simulink library "MFBD_lib"  (R2013a)
settings: Solver=ode45  StartTime=0.0  StopTime=10.0  RelTol=1e-3
values from neighbouring files (symbols this model uses):
  DPa0 = 'NA'    [getDataFromNASTRAN.m]
  EV_C = 0    [getDataFromNASTRAN.m]
  LS = 0    [getDataFromNASTRAN.m]
  omega = 0    [getDataFromNASTRAN.m]
  zeta = 'Inf'    [getDataFromNASTRAN.m]
undefined symbols (not defined in the file or in its folder): uev, uls, uw
undefined symbols (not defined in the file): ureal
libraries: RCTblocks x11, cstblocks x2
settings Model: Creator=d.alazard  LastModifiedBy=d.alazard

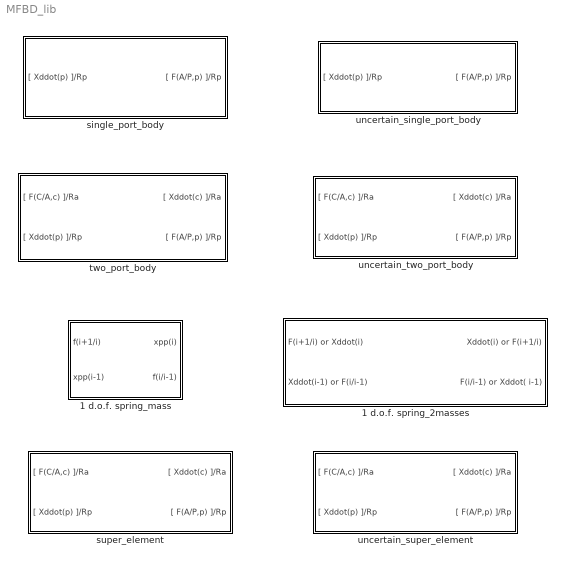
== system MFBD_lib ==
  1 d.o.f. spring_2masses : Subsystem  AncestorBlock=MFBD_lib/super_element  mask{m1=1, m2=1, k=1, c=Direct}
      mask prompts: m1 "Upstream mass: m1 (Kg)"; m2 "Downstream mass: m2 (Kg)"; k "Stiffness: k (N/m)"; c "Direct or Inverse"
      mask init:
      | path(path,'..')
      | if c==1,
      |     MKmodel=Z_elem(m1,k,m2,'d');
      | elseif c==2,
      |     MKmodel=Z_elem(m1,k,m2,'i');
      | elseif c==3,
      |     MKmodel=Z_elem(m1,k,m2,'iu');
      | elseif c==4,
      |     MKmodel=Z_elem(m1,k,m2,'il');
      | end
      mask TypeOptions c: Direct | Inverse | Upper inverse | Lower Inverse
  1 d.o.f. spring_mass : Subsystem  mask{m=0.1, k=2}
      mask prompts: m "Mass"; k "Stiffness"
  "single_port_body " : Subsystem  mask{R_angval=[0 0 0], R_sequence=ZYX, Xi=0, p_gp=1, nf=2, fbdf=file_name, ff06=file_name}
      mask prompts: R_angval "Rotation angles for appendage reference frame at P with respect to parent reference frame"; R_sequence "Rotation sequence for appendage reference frame at P"; Xi "Damping ratio for appendage"; p_gp "Grid point index corresponding to point P of appendage"; nf "No. of modes to be considered"; fbdf "Name of the .bdf file (without extension)"; ff06 "Name of the .f06 file (without extension)"
      mask init:
      | maskStr = get_param(gcb,'MaskValues');
      | R_angrad = R_angval*pi/180;
      | R_seqstr = maskStr{2};
      | dcm_au = angle2dcm(R_angrad(1),R_angrad(2),R_angrad(3),R_seqstr);
      | path(path,'..')
      | a=char(strcat(maskStr{7},'.f06'));
      | b=char(strcat(maskStr{6},'.bdf'));
      | [M, J, xcg, LS, omega, EV_C, zeta, DPa0, cdP, cdC, flagFatal] = ... 
      |     getDataFromNASTRAN(a,b,'f',Xi,p_gp,p_gp,nf);
      mask TypeOptions R_sequence: ZYX | ZYZ | ZXY | ZXZ | YXZ | YXY | YZX | YZY | XYZ | XYX | XZY | XZX
  super_element : Subsystem  AncestorBlock=MFBD_lib/super_element  mask{rho=1, s=1, l1=1, e=1, nu=1, iz=1, iy=1, ipx=1, xi=1, R_angval=[0 0 0], R_sequence=ZYX}
      mask prompts: rho "Material density, rho (kg/m^3)"; s "Beam section area, S (m^2)"; l1 "Length of the beam, L (m)"; e "Modulus of elasticity, E (Pa or N/m^2)"; nu "Poisson's ratio (Range: 0 to 0.5)"; iz "Area moment of inertia along z axis, Izz (m^4)"; iy "Area moment of inertia along y axis, Iyy (m^4)"; ipx "Polar second moment of inertia, Ipx (m^4)"; xi "Damping ratio, xi"; R_angval "Rotation angles for element reference frame at P with respect to parent reference frame"; R_sequence "Rotation sequence for element reference frame at P"
      mask init:
      | maskStr = get_param(gcb,'MaskValues');
      | R_angrad = R_angval*pi/180;
      | R_seqstr = maskStr{11};
      | dcm_eu = angle2dcm(R_angrad(1),R_angrad(2),R_angrad(3),R_seqstr);
      | g=e/(2*(1+nu));
      | path(path,'..')
      | Mm1M=TwoPortBeam(rho,s,l1,e,g,iz,iy,ipx,xi);
      mask TypeOptions R_sequence: ZYX | ZYZ | ZXY | ZXZ | YXZ | YXY | YZX | YZY | XYZ | XYX | XZY | XZX
  two_port_body : Subsystem  mask{R_angval=[0 0 0], R_sequence=ZYX, Xi=0, p_gp=1, C_gp=1, nf=2, fbdf=file_name, ff06=file_name}
      mask prompts: R_angval "Rotation angles for appendage reference frame at P with respect to parent reference frame"; R_sequence "Rotation sequence for appendage reference frame at P"; Xi "Damping ratio for appendage"; p_gp "Grid point index corresponding to point P of appendage"; C_gp "Grid point index corresponding to point C of appendage"; nf "No of modes"; fbdf "Name of the .bdf file (without extension)"; ff06 "Name of the .f06 file (without extension)"
      mask init:
      | maskStr = get_param(gcb,'MaskValues');
      | R_angrad = R_angval*pi/180;
      | R_seqstr = maskStr{2};
      | dcm_au = angle2dcm(R_angrad(1),R_angrad(2),R_angrad(3),R_seqstr);
      | path(path,'..')
      | a=char(strcat(maskStr{8},'.f06'));
      | b=char(strcat(maskStr{7},'.bdf'));
      | [M, J, xcg, LS, omega, EV_C, zeta, DPa0, cdP, cdC, flagFatal] = ... 
      |     getDataFromNASTRAN(a,b,'f',Xi,p_gp,C_gp,nf);
      | 
      | CPvec=cdP-cdC;
      | tauCP=[eye(3) [0 -CPvec(3) CPvec(2);
      |                CPvec(3) 0 -CPvec(1);
      |               -CPvec(2) CPvec(1) 0];
      |               zeros(3) eye(3)];
      mask TypeOptions R_sequence: ZYX | ZYZ | ZXY | ZXZ | YXZ | YXY | YZX | YZY | XYZ | XYX | XZY | XZX
  uncertain_single_port_body : Subsystem  mask{R_angval=[0 0 0], R_sequence=ZYX, Xi=0, p_gp=1, uw_var=0, uls_var=0, nf=2, fbdf=file_name, ff06=file_name}
      mask prompts: R_angval "Rotation angles for appendage reference frame at P with respect to parent reference frame"; R_sequence "Rotation sequence for appendage reference frame at P"; Xi "Damping ratio for appendage"; p_gp "Grid point index corresponding to point P of appendage"; uw_var "Percentage of uncertainity for natural frequencies"; uls_var "Percentage of uncertainity for modal participation factors"; nf "Number of modes"; fbdf "Name of the .bdf file (without extension)"; ff06 "Name of the .f06 file (without extension)"
      mask init:
      | maskStr = get_param(gcb,'MaskValues');
      | R_angrad = R_angval*pi/180;
      | R_seqstr = maskStr{2};
      | dcm_au = angle2dcm(R_angrad(1),R_angrad(2),R_angrad(3),R_seqstr);
      | path(path,'..')
      | a=char(strcat(maskStr{9},'.f06'));
      | b=char(strcat(maskStr{8},'.bdf'));
      | [M, J, xcg, LS, omega, EV_C, zeta, DPa0, cdP, cdC, flagFatal] = ... 
      |     getDataFromNASTRAN(a,b,'f',Xi,p_gp,p_gp,nf);
      | for i=1:size(omega)
      |     uw(i)=eval(['ureal(''uwa' num2str(i) ''',' num2str(omega(i)) ... 
      |         ',''Percentage'',' num2str(uw_var) ')' ]);
      | end
      | 
      | sLS=size(LS);
      | 
      | for i=1:sLS(1)
      |     for j=1:sLS(2)
      |         if(LS(i,j)==0)
      |             uls(i,j)=0;
      |         else
      |         uls(i,j)=eval(['ureal(''ulsa' num2str(i) num2str(j) ''',' num2str(LS(i,j)) ... 
      |         ',''Percentage'',' num2str(uls_var) ')' ]);
      |         end
      |     end
      | end
      mask TypeOptions R_sequence: ZYX | ZYZ | ZXY | ZXZ | YXZ | YXY | YZX | YZY | XYZ | XYX | XZY | XZX
  uncertain_super_element : Subsystem  AncestorBlock=MFBD_lib/super_element  mask{rho=ureal('rho',1,'Percentage',1), s=ureal('S',1,'Percentage',1), l1=ureal('L',1,'Percentage',1), e=ureal('E',1,'Percentage',1), nu=ureal('nu',0.3,'Percentage',1), iz=ureal('Izz',1,'Percentage',1), iy=ureal('Iyy',1,'Percentage',1), ipx=ureal('Ipx',1,'Percentage',1), xi=ureal('xi',1,'Percentage',1), R_angval=[0 0 0], R_sequence=ZYX}
      mask prompts: rho "Material density, rho (kg/m^3)"; s "Beam section area, S (m^2)"; l1 "Length of the beam, L (m)"; e "Modulus of elasticity, E (Pa or N/m^2)"; nu "Poisson's ratio (Range: 0 to 0.5)"; iz "Area moment of inertia along z axis, Izz (m^4)"; iy "Area moment of inertia along y axis, Iyy (m^4)"; ipx "Polar second moment of inertia, Ipx (m^4)"; xi "Damping ratio, xi"; R_angval "Rotation angles for element reference frame at P with respect to parent reference frame"; R_sequence "Rotation sequence for element reference frame at P"
      mask init:
      | maskStr = get_param(gcb,'MaskValues');
      | R_angrad = R_angval*pi/180;
      | R_seqstr = maskStr{11};
      | dcm_eu = angle2dcm(R_angrad(1),R_angrad(2),R_angrad(3),R_seqstr);
      | path(path,'..')
      | g=e/(2*(1+nu));
      | Mm1M=TwoPortBeam(rho,s,l1,e,g,iz,iy,ipx,xi);
      mask TypeOptions R_sequence: ZYX | ZYZ | ZXY | ZXZ | YXZ | YXY | YZX | YZY | XYZ | XYX | XZY | XZX
  uncertain_two_port_body : Subsystem  mask{R_angval=[0 0 0], R_sequence=ZYX, Xi=0, p_gp=1, C_gp=1, uw_var=0, uev_var=0, uls_var=0, nf=2, fbdf=file_name, ff06=file_name}
      mask prompts: R_angval "Rotation angles for appendage reference frame at P with respect to parent reference frame"; R_sequence "Rotation sequence for appendage reference frame at P"; Xi "Damping ratio for appendage"; p_gp "Grid point index corresponding to point P of appendage"; C_gp "Grid point index corresponding to point C of appendage"; uw_var "Percentage of uncertainity for natural frequencies"; uev_var "Percentage of uncertainity for Eigen vectors"; uls_var "Percentage of uncertainity for modal participation factors"; nf "No. of modes"; fbdf "Name of the .bdf file (without extension)"; ff06 "Name of the .f06 file (without extension)"
      mask init:
      | maskStr = get_param(gcb,'MaskValues');
      | R_angrad = R_angval*pi/180;
      | R_seqstr = maskStr{2};
      | dcm_au = angle2dcm(R_angrad(1),R_angrad(2),R_angrad(3),R_seqstr);
      | path(path,'..')
      | a=char(strcat(maskStr{11},'.f06'));
      | b=char(strcat(maskStr{10},'.bdf'));
      | [M, J, xcg, LS, omega, EV_C, zeta, DPa0, cdP, cdC, flagFatal] = ... 
      |     getDataFromNASTRAN(a,b,'f',Xi,p_gp,C_gp,nf);
      | 
      | CPvec=cdP-cdC;
      | tauCP=[eye(3) [0 -CPvec(3) CPvec(2);
      |                CPvec(3) 0 -CPvec(1);
      |               -CPvec(2) CPvec(1) 0];
      |               zeros(3) eye(3)];
      | 
      | for i=1:size(omega)
      |     uw(i)=eval(['ureal(''uwa' num2str(i) ''',' num2str(omega(i)) ... 
      |         ',''Percentage'',' num2str(uw_var) ')' ]);
      | end
      | 
      | sLS=size(LS);
      | sEV=size(EV_C);
      | 
      | for i=1:sLS(1)
      |     for j=1:sLS(2)
      |         if(LS(i,j)==0)
      |             uls(i,j)=0;
      |         else
      |         uls(i,j)=eval(['ureal(''ulsa' num2str(i) num2str(j) ''',' num2str(LS(i,j)) ... 
      |         ',''Percentage'',' num2str(uls_var) ')' ]);
      |         end
      |     end
      | end
      | 
      | for i=1:sEV(1)
      |     for j=1:sEV(2)
      |         if(EV_C(i,j)==0)
      |             uev(i,j)=0;
      |         else
      |         uev(i,j)=eval(['ureal(''ueva' num2str(i) num2str(j) ''',' num2str(EV_C(i,j)) ... 
      |         ',''Percentage'',' num2str(uev_var) ')' ]);
      |         end
      |     end
      | end
      mask TypeOptions R_sequence: ZYX | ZYZ | ZXY | ZXZ | YXZ | YXY | YZX | YZY | XYZ | XYX | XZY | XZX

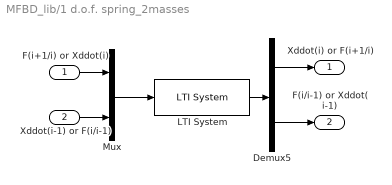
== system MFBD_lib/1 d.o.f. spring_2masses ==
  F(i+1/i) or Xddot(i) : Inport
  Xddot(i-1) or F(i/i-1) : Inport  Port=2
  Demux5 : Demux  Outputs=2
  LTI System : cstblocks/LTI System  sys=MKmodel  IC=[]
  Mux : Mux  Inputs=2
  Xddot(i) or F(i+1/i) : Outport
  F(i/i-1) or Xddot( i-1) : Outport  Port=2
  wires:
  Mux/1 -> LTI System/1
  LTI System/1 -> Demux5/1
  F(i+1/i) or Xddot(i)/1 -> Mux/1
  Xddot(i-1) or F(i/i-1)/1 -> Mux/2
  Demux5/1 -> Xddot(i) or F(i+1/i)/1
  Demux5/2 -> F(i/i-1) or Xddot( i-1)/1

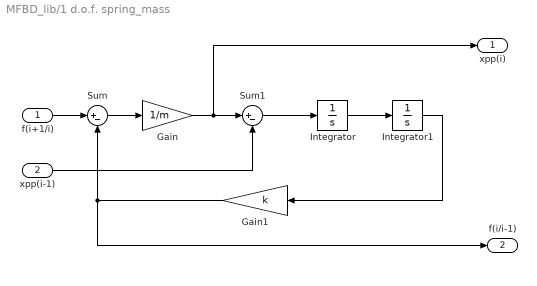
== system MFBD_lib/1 d.o.f. spring_mass ==
  f(i+1/i) : Inport
  xpp(i-1) : Inport  Port=2
  Gain : Gain  Gain=1/m
  Gain1 : Gain  Gain=k
  Integrator : Integrator
  Integrator1 : Integrator
  Sum : Sum  Inputs=|+-
  Sum1 : Sum  Inputs=|+-
  xpp(i) : Outport
  f(i/i-1) : Outport  Port=2
  wires:
  xpp(i-1)/1 -> Sum1/2
  f(i+1/i)/1 -> Sum/1
  Integrator1/1 -> Gain1/1
  Sum1/1 -> Integrator/1
  Integrator/1 -> Integrator1/1
  Sum/1 -> Gain/1
  Gain/1 -> xpp(i)/1, Sum1/1
  Gain1/1 -> f(i/i-1)/1, Sum/2

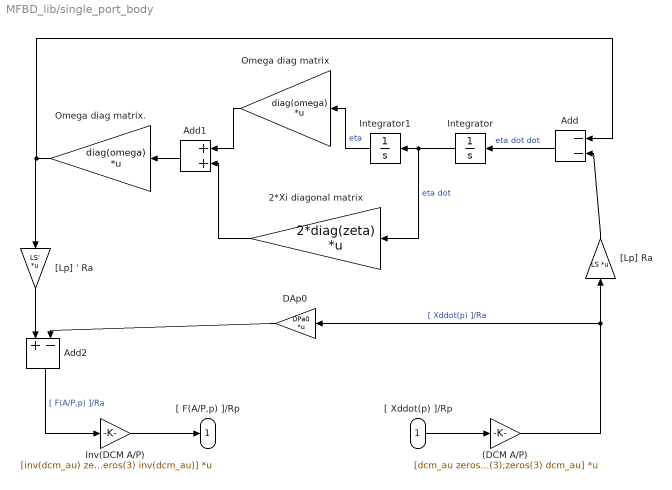
== system MFBD_lib/single_port_body  ==
  "[ Xddot(p) ]/Rp" : Inport
  (DCM A/P) : Gain  Gain=[dcm_au zeros(3);zeros(3) dcm_au]  Multiplication=Matrix(K*u)
  2*Xi diagonal matrix : Gain  Gain=2*diag(zeta)  Multiplication=Matrix(K*u)
  Add : Sum  Inputs=--
  Add1 : Sum
  Add2 : Sum  Inputs=+-
  DAp0 : Gain  Gain=DPa0  Multiplication=Matrix(K*u)
  Integrator : Integrator
  Integrator1 : Integrator
  Inv(DCM A/P) : Gain  Gain=[inv(dcm_au) zeros(3);zeros(3) inv(dcm_au)]  Multiplication=Matrix(K*u)
  Omega diag matrix : Gain  Gain=diag(omega)  Multiplication=Matrix(K*u)
  Omega diag matrix. : Gain  Gain=diag(omega)  Multiplication=Matrix(K*u)
  "[Lp] ' Ra" : Gain  Gain=LS'  Multiplication=Matrix(K*u)
  "[Lp] Ra" : Gain  Gain=LS  Multiplication=Matrix(K*u)
  "[ F(A/P,p) ]/Rp" : Outport
  wires:
  Add2/1 -> Inv(DCM A/P)/1  "[ F(A/P,p) ]/Ra"
  Inv(DCM A/P)/1 -> "[ F(A/P,p) ]/Rp"/1
  Omega diag matrix./1 -> Add/1, "[Lp] ' Ra"/1
  "[Lp] Ra"/1 -> Add/2
  2*Xi diagonal matrix/1 -> Add1/2
  Add1/1 -> Omega diag matrix./1
  Add/1 -> Integrator/1  "eta dot dot"
  Integrator1/1 -> Omega diag matrix/1  "eta"
  "[ Xddot(p) ]/Rp"/1 -> (DCM A/P)/1
  Integrator/1 -> 2*Xi diagonal matrix/1, Integrator1/1  "eta dot"
  Omega diag matrix/1 -> Add1/1
  (DCM A/P)/1 -> "[Lp] Ra"/1, DAp0/1  "[ Xddot(p) ]/Ra"
  "[Lp] ' Ra"/1 -> Add2/1
  DAp0/1 -> Add2/2

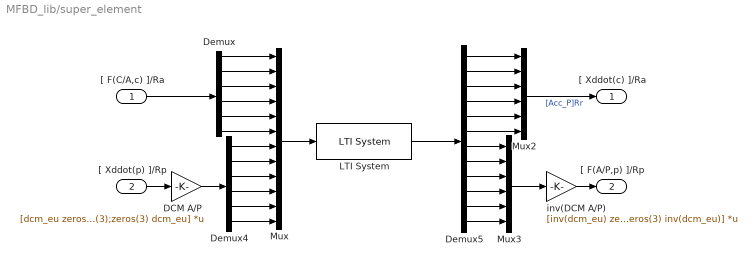
== system MFBD_lib/super_element ==
  "[ F(C/A,c) ]/Ra" : Inport
  "[ Xddot(p) ]/Rp" : Inport  Port=2
  DCM A/P : Gain  Gain=[dcm_eu zeros(3);zeros(3) dcm_eu]  Multiplication=Matrix(K*u)
  Demux : Demux  Outputs=6
  Demux4 : Demux  Outputs=6
  Demux5 : Demux  Outputs=12
  LTI System : cstblocks/LTI System  sys=Mm1M  IC=[]
  Mux : Mux  Inputs=12
  Mux2 : Mux  Inputs=6
  Mux3 : Mux  Inputs=6
  inv(DCM A/P) : Gain  Gain=[inv(dcm_eu) zeros(3);zeros(3) inv(dcm_eu)]  Multiplication=Matrix(K*u)
  "[ Xddot(c) ]/Ra" : Outport
  "[ F(A/P,p) ]/Rp" : Outport  Port=2
  wires:
  Demux5/8 -> Mux3/2
  Mux/1 -> LTI System/1
  Demux5/9 -> Mux3/3
  Demux4/5 -> Mux/11
  Demux4/3 -> Mux/9
  Demux5/7 -> Mux3/1
  Demux/2 -> Mux/2
  "[ Xddot(p) ]/Rp"/1 -> DCM A/P/1
  Mux2/1 -> "[ Xddot(c) ]/Ra"/1  "[Acc_P]Rr"
  Demux/3 -> Mux/3
  LTI System/1 -> Demux5/1
  Mux3/1 -> inv(DCM A/P)/1
  Demux/6 -> Mux/6
  Demux4/2 -> Mux/8
  Demux5/1 -> Mux2/1
  Demux5/12 -> Mux3/6
  Demux5/5 -> Mux2/5
  Demux5/11 -> Mux3/5
  Demux4/6 -> Mux/12
  Demux4/1 -> Mux/7
  Demux5/2 -> Mux2/2
  Demux5/6 -> Mux2/6
  Demux5/3 -> Mux2/3
  Demux/4 -> Mux/4
  Demux5/4 -> Mux2/4
  "[ F(C/A,c) ]/Ra"/1 -> Demux/1
  Demux4/4 -> Mux/10
  DCM A/P/1 -> Demux4/1
  Demux/5 -> Mux/5
  Demux5/10 -> Mux3/4
  Demux/1 -> Mux/1
  inv(DCM A/P)/1 -> "[ F(A/P,p) ]/Rp"/1

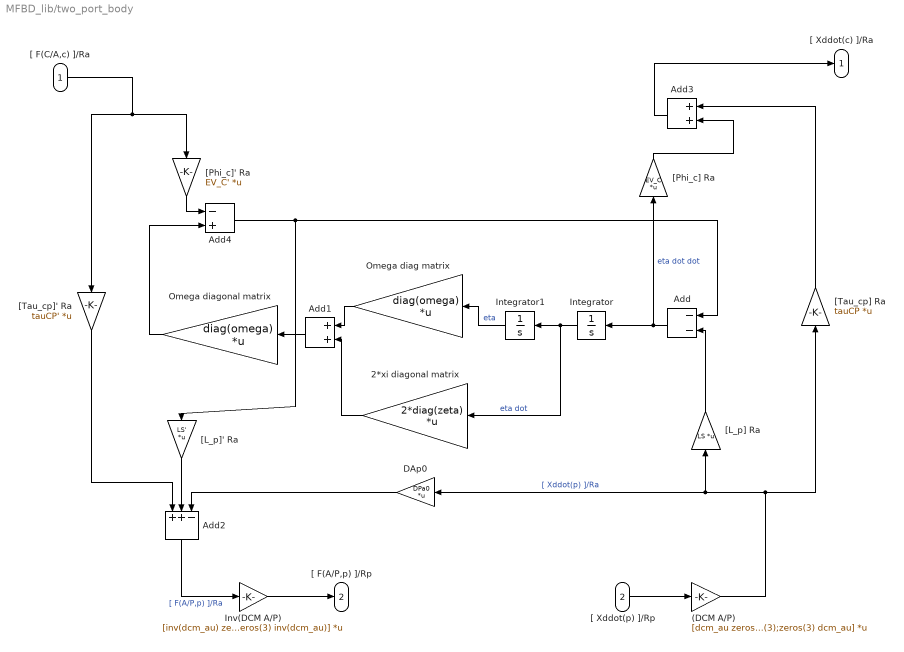
== system MFBD_lib/two_port_body ==
  "[ F(C/A,c) ]/Ra" : Inport
  "[ Xddot(p) ]/Rp" : Inport  Port=2
  (DCM A/P) : Gain  Gain=[dcm_au zeros(3);zeros(3) dcm_au]  Multiplication=Matrix(K*u)
  2*xi diagonal matrix : Gain  Gain=2*diag(zeta)  Multiplication=Matrix(K*u) (u vector)
  Add : Sum  Inputs=--
  Add1 : Sum
  Add2 : Sum  Inputs=++-
  Add3 : Sum
  Add4 : Sum  Inputs=-+
  DAp0 : Gain  Gain=DPa0  Multiplication=Matrix(K*u)
  Integrator : Integrator
  Integrator1 : Integrator
  Inv(DCM A/P) : Gain  Gain=[inv(dcm_au) zeros(3);zeros(3) inv(dcm_au)]  Multiplication=Matrix(K*u)
  Omega diag matrix : Gain  Gain=diag(omega)  Multiplication=Matrix(K*u) (u vector)
  Omega diagonal matrix : Gain  Gain=diag(omega)  Multiplication=Matrix(K*u) (u vector)
  "[L_p] Ra" : Gain  Gain=LS  Multiplication=Matrix(K*u)
  "[L_p]' Ra" : Gain  Gain=LS'  Multiplication=Matrix(K*u)
  "[Phi_c] Ra" : Gain  Gain=EV_C  Multiplication=Matrix(K*u)
  "[Phi_c]' Ra" : Gain  Gain=EV_C'  Multiplication=Matrix(K*u)
  "[Tau_cp] Ra" : Gain  Gain=tauCP  Multiplication=Matrix(K*u)
  "[Tau_cp]' Ra" : Gain  Gain=tauCP'  Multiplication=Matrix(K*u)
  "[ Xddot(c) ]/Ra" : Outport
  "[ F(A/P,p) ]/Rp" : Outport  Port=2
  wires:
  Add2/1 -> Inv(DCM A/P)/1  "[ F(A/P,p) ]/Ra"
  Inv(DCM A/P)/1 -> "[ F(A/P,p) ]/Rp"/1
  "[ F(C/A,c) ]/Ra"/1 -> "[Phi_c]' Ra"/1, "[Tau_cp]' Ra"/1
  Add4/1 -> Add/1, "[L_p]' Ra"/1
  "[Phi_c]' Ra"/1 -> Add4/1
  Add3/1 -> "[ Xddot(c) ]/Ra"/1
  "[Phi_c] Ra"/1 -> Add3/2
  "[Tau_cp] Ra"/1 -> Add3/1
  "[L_p] Ra"/1 -> Add/2
  2*xi diagonal matrix/1 -> Add1/2
  Add1/1 -> Omega diagonal matrix/1
  Add/1 -> Integrator/1, "[Phi_c] Ra"/1  "eta dot dot"
  Integrator1/1 -> Omega diag matrix/1  "eta"
  "[ Xddot(p) ]/Rp"/1 -> (DCM A/P)/1
  Integrator/1 -> Integrator1/1, 2*xi diagonal matrix/1  "eta dot"
  Omega diag matrix/1 -> Add1/1
  Omega diagonal matrix/1 -> Add4/2
  (DCM A/P)/1 -> "[Tau_cp] Ra"/1, "[L_p] Ra"/1, DAp0/1  "[ Xddot(p) ]/Ra"
  DAp0/1 -> Add2/3
  "[L_p]' Ra"/1 -> Add2/2
  "[Tau_cp]' Ra"/1 -> Add2/1

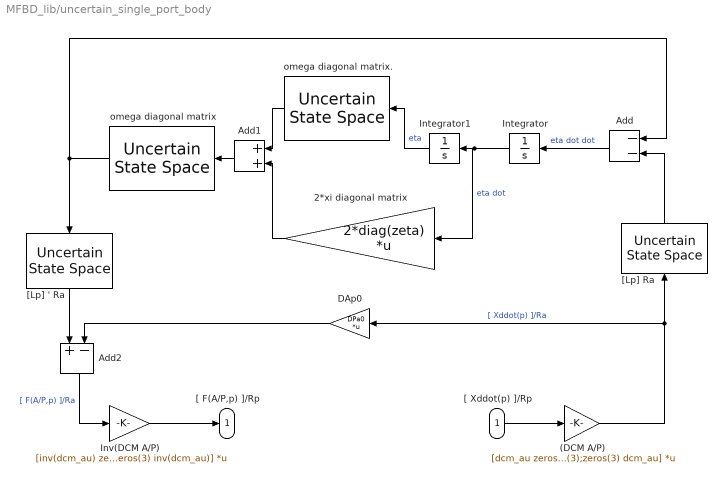
== system MFBD_lib/uncertain_single_port_body ==
  "[ Xddot(p) ]/Rp" : Inport
  (DCM A/P) : Gain  Gain=[dcm_au zeros(3);zeros(3) dcm_au]  Multiplication=Matrix(K*u)
  2*xi diagonal matrix : Gain  Gain=2*diag(zeta)  Multiplication=Matrix(K*u) (u vector)
  Add : Sum  Inputs=--
  Add1 : Sum
  Add2 : Sum  Inputs=+-
  DAp0 : Gain  Gain=DPa0  Multiplication=Matrix(K*u)
  Integrator : Integrator
  Integrator1 : Integrator
  Inv(DCM A/P) : Gain  Gain=[inv(dcm_au) zeros(3);zeros(3) inv(dcm_au)]  Multiplication=Matrix(K*u)
  "[Lp] ' Ra" : RCTblocks/Uncertain State Space  Tag=USS  USystem=ss([],[],[],uls')  UValue=[]  X0=[]  uX0=[]
  "[Lp] Ra" : RCTblocks/Uncertain State Space  Tag=USS  USystem=ss([],[],[],uls)  UValue=[]  X0=[]  uX0=[]
  omega diagonal matrix : RCTblocks/Uncertain State Space  Tag=USS  USystem=ss([],[],[],diag(uw))  UValue=[]  X0=[]  uX0=[]
  omega diagonal matrix. : RCTblocks/Uncertain State Space  Tag=USS  USystem=ss([],[],[],diag(uw))  UValue=[]  X0=[]  uX0=[]
  "[ F(A/P,p) ]/Rp" : Outport
  wires:
  Add2/1 -> Inv(DCM A/P)/1  "[ F(A/P,p) ]/Ra"
  Inv(DCM A/P)/1 -> "[ F(A/P,p) ]/Rp"/1
  omega diagonal matrix/1 -> Add/1, "[Lp] ' Ra"/1
  "[Lp] Ra"/1 -> Add/2
  2*xi diagonal matrix/1 -> Add1/2
  Add1/1 -> omega diagonal matrix/1
  Add/1 -> Integrator/1  "eta dot dot"
  Integrator1/1 -> omega diagonal matrix./1  "eta"
  "[ Xddot(p) ]/Rp"/1 -> (DCM A/P)/1
  Integrator/1 -> 2*xi diagonal matrix/1, Integrator1/1  "eta dot"
  omega diagonal matrix./1 -> Add1/1
  (DCM A/P)/1 -> DAp0/1, "[Lp] Ra"/1  "[ Xddot(p) ]/Ra"
  "[Lp] ' Ra"/1 -> Add2/1
  DAp0/1 -> Add2/2

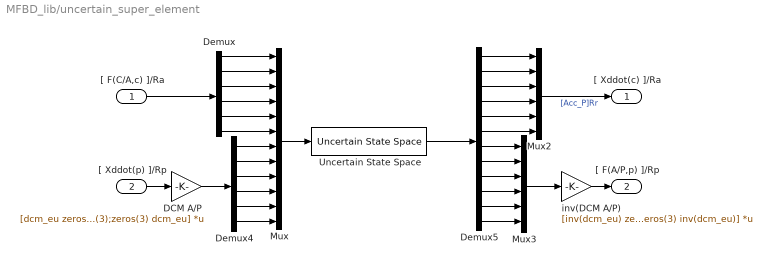
== system MFBD_lib/uncertain_super_element ==
  "[ F(C/A,c) ]/Ra" : Inport
  "[ Xddot(p) ]/Rp" : Inport  Port=2
  DCM A/P : Gain  Gain=[dcm_eu zeros(3);zeros(3) dcm_eu]  Multiplication=Matrix(K*u)
  Demux : Demux  Outputs=6
  Demux4 : Demux  Outputs=6
  Demux5 : Demux  Outputs=12
  Mux : Mux  Inputs=12
  Mux2 : Mux  Inputs=6
  Mux3 : Mux  Inputs=6
  Uncertain State Space : RCTblocks/Uncertain State Space  Tag=USS  USystem=Mm1M  UValue=[]  X0=[]  uX0=[]
  inv(DCM A/P) : Gain  Gain=[inv(dcm_eu) zeros(3);zeros(3) inv(dcm_eu)]  Multiplication=Matrix(K*u)
  "[ Xddot(c) ]/Ra" : Outport
  "[ F(A/P,p) ]/Rp" : Outport  Port=2
  wires:
  Mux/1 -> Uncertain State Space/1
  Demux4/5 -> Mux/11
  Demux4/3 -> Mux/9
  Demux/2 -> Mux/2
  "[ Xddot(p) ]/Rp"/1 -> DCM A/P/1
  Demux/3 -> Mux/3
  Demux/6 -> Mux/6
  Demux4/2 -> Mux/8
  Demux4/6 -> Mux/12
  Demux4/1 -> Mux/7
  Demux/4 -> Mux/4
  "[ F(C/A,c) ]/Ra"/1 -> Demux/1
  Demux4/4 -> Mux/10
  DCM A/P/1 -> Demux4/1
  Demux/5 -> Mux/5
  Demux/1 -> Mux/1
  Demux5/8 -> Mux3/2
  Demux5/9 -> Mux3/3
  Demux5/7 -> Mux3/1
  Mux2/1 -> "[ Xddot(c) ]/Ra"/1  "[Acc_P]Rr"
  Uncertain State Space/1 -> Demux5/1
  Mux3/1 -> inv(DCM A/P)/1
  Demux5/1 -> Mux2/1
  Demux5/12 -> Mux3/6
  Demux5/5 -> Mux2/5
  Demux5/11 -> Mux3/5
  Demux5/2 -> Mux2/2
  Demux5/6 -> Mux2/6
  Demux5/3 -> Mux2/3
  Demux5/4 -> Mux2/4
  Demux5/10 -> Mux3/4
  inv(DCM A/P)/1 -> "[ F(A/P,p) ]/Rp"/1

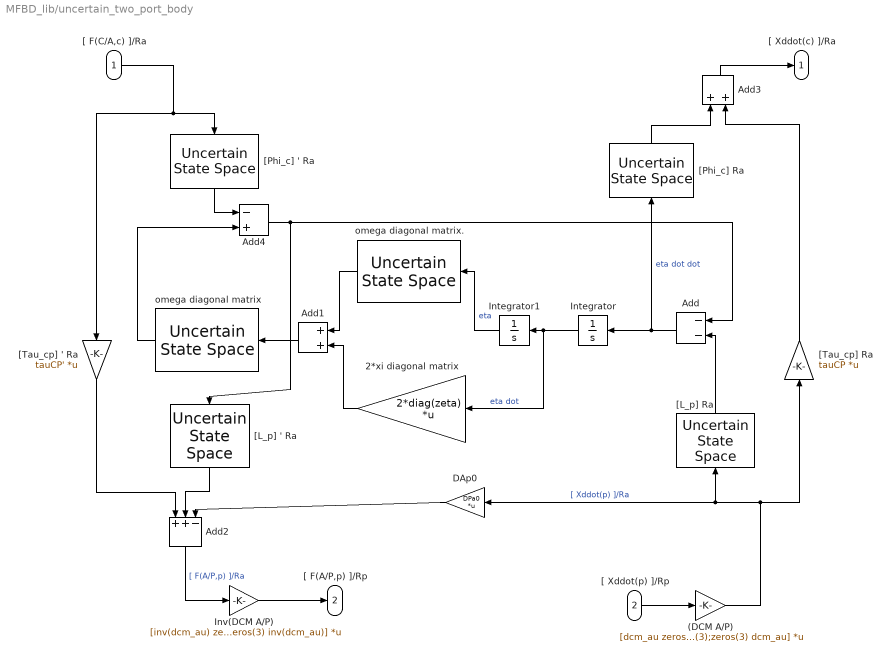
== system MFBD_lib/uncertain_two_port_body ==
  "[ F(C/A,c) ]/Ra" : Inport
  "[ Xddot(p) ]/Rp" : Inport  Port=2
  (DCM A/P) : Gain  Gain=[dcm_au zeros(3);zeros(3) dcm_au]  Multiplication=Matrix(K*u)
  2*xi diagonal matrix : Gain  Gain=2*diag(zeta)  Multiplication=Matrix(K*u) (u vector)
  Add : Sum  Inputs=--
  Add1 : Sum
  Add2 : Sum  Inputs=++-
  Add3 : Sum
  Add4 : Sum  Inputs=-+
  DAp0 : Gain  Gain=DPa0  Multiplication=Matrix(K*u)
  Integrator : Integrator
  Integrator1 : Integrator
  Inv(DCM A/P) : Gain  Gain=[inv(dcm_au) zeros(3);zeros(3) inv(dcm_au)]  Multiplication=Matrix(K*u)
  "[L_p] ' Ra" : RCTblocks/Uncertain State Space  Tag=USS  USystem=ss([],[],[],uls')  UValue=[]  X0=[]  uX0=[]
  "[L_p] Ra" : RCTblocks/Uncertain State Space  Tag=USS  USystem=ss([],[],[],uls)  UValue=[]  X0=[]  uX0=[]
  "[Phi_c] ' Ra" : RCTblocks/Uncertain State Space  Tag=USS  USystem=ss([],[],[],uev')  UValue=[]  X0=[]  uX0=[]
  "[Phi_c] Ra" : RCTblocks/Uncertain State Space  Tag=USS  USystem=ss([],[],[],uev)  UValue=[]  X0=[]  uX0=[]
  "[Tau_cp] ' Ra" : Gain  Gain=tauCP'  Multiplication=Matrix(K*u)
  "[Tau_cp] Ra" : Gain  Gain=tauCP  Multiplication=Matrix(K*u)
  omega diagonal matrix : RCTblocks/Uncertain State Space  Tag=USS  USystem=ss([],[],[],diag(uw))  UValue=[]  X0=[]  uX0=[]
  omega diagonal matrix. : RCTblocks/Uncertain State Space  Tag=USS  USystem=ss([],[],[],diag(uw))  UValue=[]  X0=[]  uX0=[]
  "[ Xddot(c) ]/Ra" : Outport
  "[ F(A/P,p) ]/Rp" : Outport  Port=2
  wires:
  Add2/1 -> Inv(DCM A/P)/1  "[ F(A/P,p) ]/Ra"
  Inv(DCM A/P)/1 -> "[ F(A/P,p) ]/Rp"/1
  "[ F(C/A,c) ]/Ra"/1 -> "[Phi_c] ' Ra"/1, "[Tau_cp] ' Ra"/1
  "[Tau_cp] ' Ra"/1 -> Add2/1
  Add4/1 -> "[L_p] ' Ra"/1, Add/1
  "[Phi_c] ' Ra"/1 -> Add4/1
  Add3/1 -> "[ Xddot(c) ]/Ra"/1
  "[L_p] Ra"/1 -> Add/2
  2*xi diagonal matrix/1 -> Add1/2
  Add1/1 -> omega diagonal matrix/1
  Add/1 -> Integrator/1, "[Phi_c] Ra"/1  "eta dot dot"
  Integrator1/1 -> omega diagonal matrix./1  "eta"
  "[ Xddot(p) ]/Rp"/1 -> (DCM A/P)/1
  Integrator/1 -> 2*xi diagonal matrix/1, Integrator1/1  "eta dot"
  omega diagonal matrix./1 -> Add1/1
  DAp0/1 -> Add2/3
  "[L_p] ' Ra"/1 -> Add2/2
  omega diagonal matrix/1 -> Add4/2
  (DCM A/P)/1 -> "[Tau_cp] Ra"/1, DAp0/1, "[L_p] Ra"/1  "[ Xddot(p) ]/Ra"
  "[Phi_c] Ra"/1 -> Add3/1
  "[Tau_cp] Ra"/1 -> Add3/2
